simulink model "q2_model"  (R2021b)
settings: Solver=VariableStepAuto  StartTime=0.0  StopTime=1000  RelTol=1e-3
undefined symbols (not defined in the file or in its folder): DiscIntNeverNeededParam
libraries: dspswit3 x1
settings Model: Creator=jeff  LastModifiedBy=jeff

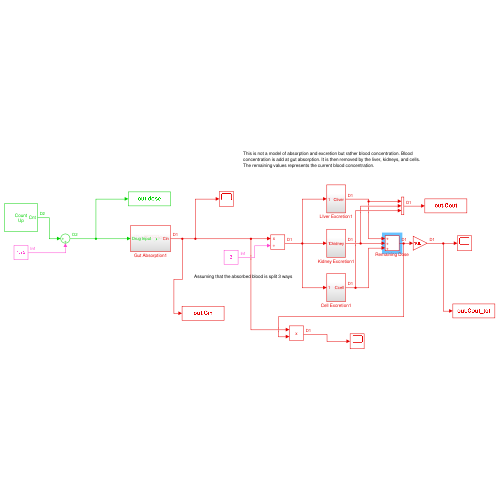
[thumbnail: Simulink's stored preview of the top-level diagram]
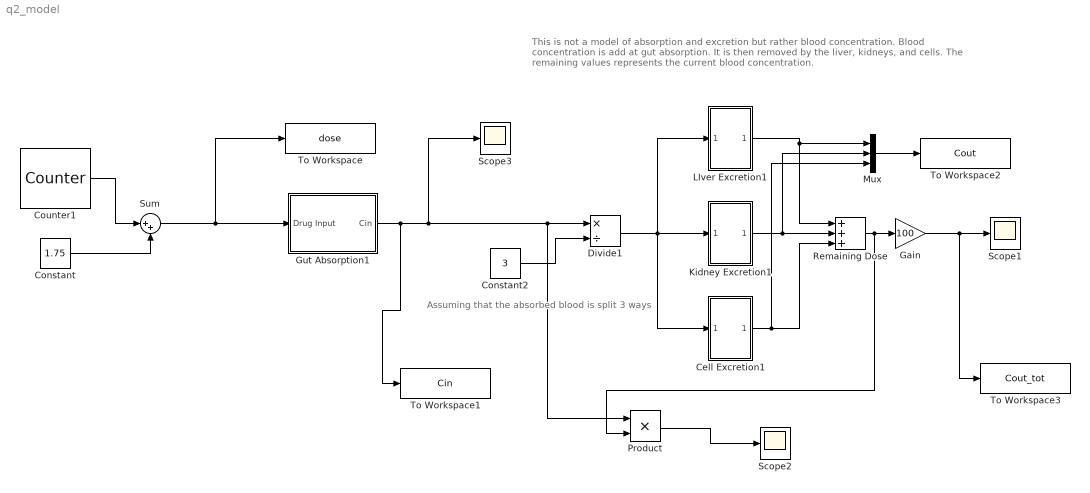
== system q2_model ==
  note: Assuming that the absorbed blood is split 3 ways
  note: This is not a model of absorption and excretion but rather blood concentration. Blood concentration is add at gut absorption. It is then removed by the liver, kidneys, and cells. The remaining values represents the current blood concentration.
  Cell Excretion1 : Subsystem
  Constant : Constant  Value=1.75
  Constant2 : Constant  Value=3
  Counter1 : dspswit3/Counter  Direction=Up  CountEvent=Free running  CounterSize=User defined  MaxCount=255  InitialCount=0  Output=Count  HitValue=32  ResetInput=off  SamplesPerFrame=1  Ts=90  CntDtype=double  HitDtype=Logical
  Divide1 : Product  Inputs=*/
  Gain : Gain  Gain=100
  Gut Absorption1 : Subsystem
  Kidney Excretion1 : Subsystem
  LIver Excretion1 : Subsystem
  Mux : Mux  Inputs=3
  Product : Product
  Remaining Dose : Sum  Inputs=+++
  Scope1 : Scope
  Scope2 : Scope
  Scope3 : Scope
  Sum : Sum  Inputs=|++
  To Workspace : ToWorkspace  VariableName=dose  SaveFormat=Timeseries  SampleTime=-1
  To Workspace1 : ToWorkspace  VariableName=Cin  SaveFormat=Timeseries  SampleTime=-1
  To Workspace2 : ToWorkspace  VariableName=Cout  SaveFormat=Timeseries  SampleTime=-1
  To Workspace3 : ToWorkspace  VariableName=Cout_tot  SaveFormat=Timeseries  SampleTime=-1
  wires:
  Constant2/1 -> Divide1/2
  Divide1/1 -> Cell Excretion1/1(In2), Kidney Excretion1/1(In1), LIver Excretion1/1(In1)
  Kidney Excretion1/1(Ckidney) -> Mux/2, Remaining Dose/2
  Cell Excretion1/1(Ccell) -> Mux/3, Remaining Dose/3
  Remaining Dose/1 -> Product/2, Gain/1
  LIver Excretion1/1(Cliver) -> Remaining Dose/1, Mux/1
  Gut Absorption1/1(Cin) -> Product/1, Divide1/1, Scope3/1, To Workspace1/1
  Counter1/1 -> Sum/1
  Mux/1 -> To Workspace2/1
  Gain/1 -> To Workspace3/1, Scope1/1
  Product/1 -> Scope2/1
  Constant/1 -> Sum/2
  Sum/1 -> To Workspace/1, Gut Absorption1/1(Drug Input)

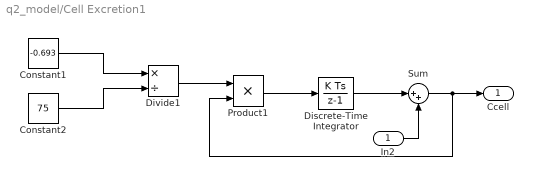
== system q2_model/Cell Excretion1 ==
  In2 : Inport
  Constant1 : Constant  Value=-0.693
  Constant2 : Constant  Value=75
  Discrete-Time Integrator : DiscreteIntegrator  SampleTime=-1  ICPrevOutput=DiscIntNeverNeededParam  ICPrevScaledInput=DiscIntNeverNeededParam
  Divide1 : Product  Inputs=*/
  Product1 : Product
  Sum : Sum  Inputs=|++
  Ccell : Outport
  wires:
  Discrete-Time Integrator/1 -> Sum/1
  Product1/1 -> Discrete-Time Integrator/1
  In2/1 -> Sum/2
  Divide1/1 -> Product1/1
  Sum/1 -> Ccell/1, Product1/2
  Constant1/1 -> Divide1/1
  Constant2/1 -> Divide1/2

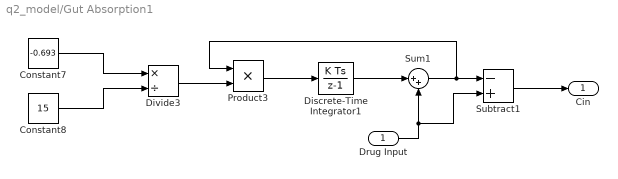
== system q2_model/Gut Absorption1 ==
  Drug Input : Inport
  Constant7 : Constant  Value=-0.693
  Constant8 : Constant  Value=15
  Discrete-Time Integrator1 : DiscreteIntegrator  SampleTime=0.1  ICPrevOutput=DiscIntNeverNeededParam  ICPrevScaledInput=DiscIntNeverNeededParam
  Divide3 : Product  Inputs=*/
  Product3 : Product
  Subtract1 : Sum  Inputs=-+
  Sum1 : Sum  Inputs=|++
  Cin : Outport
  wires:
  Discrete-Time Integrator1/1 -> Sum1/1
  Product3/1 -> Discrete-Time Integrator1/1
  Sum1/1 -> Product3/1, Subtract1/1
  Constant7/1 -> Divide3/1
  Constant8/1 -> Divide3/2
  Drug Input/1 -> Sum1/2, Subtract1/2
  Subtract1/1 -> Cin/1
  Divide3/1 -> Product3/2

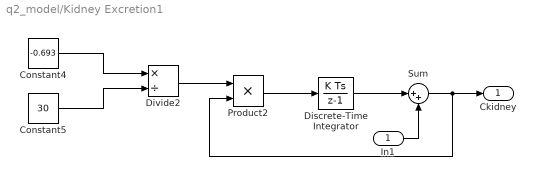
== system q2_model/Kidney Excretion1 ==
  In1 : Inport
  Constant4 : Constant  Value=-0.693
  Constant5 : Constant  Value=30
  Discrete-Time Integrator : DiscreteIntegrator  SampleTime=-1  ICPrevOutput=DiscIntNeverNeededParam  ICPrevScaledInput=DiscIntNeverNeededParam
  Divide2 : Product  Inputs=*/
  Product2 : Product
  Sum : Sum  Inputs=|++
  Ckidney : Outport
  wires:
  Discrete-Time Integrator/1 -> Sum/1
  Product2/1 -> Discrete-Time Integrator/1
  In1/1 -> Sum/2
  Divide2/1 -> Product2/1
  Sum/1 -> Ckidney/1, Product2/2
  Constant4/1 -> Divide2/1
  Constant5/1 -> Divide2/2

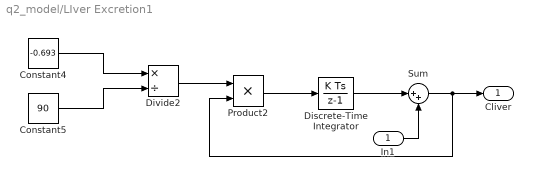
== system q2_model/LIver Excretion1 ==
  In1 : Inport
  Constant4 : Constant  Value=-0.693
  Constant5 : Constant  Value=90
  Discrete-Time Integrator : DiscreteIntegrator  SampleTime=-1  ICPrevOutput=DiscIntNeverNeededParam  ICPrevScaledInput=DiscIntNeverNeededParam
  Divide2 : Product  Inputs=*/
  Product2 : Product
  Sum : Sum  Inputs=|++
  Cliver : Outport
  wires:
  Divide2/1 -> Product2/1
  Constant5/1 -> Divide2/2
  Constant4/1 -> Divide2/1
  Product2/1 -> Discrete-Time Integrator/1
  Discrete-Time Integrator/1 -> Sum/1
  In1/1 -> Sum/2
  Sum/1 -> Cliver/1, Product2/2
